simulink model "SHARIEF3IC"  (Simulink 6.6)
settings: Solver=ode45  StartTime=0.0  StopTime=0.01  RelTol=1e-3
libraries: powerlib x10
settings Model: Creator=Y9EE1238  LastModifiedBy=Y9EE1238

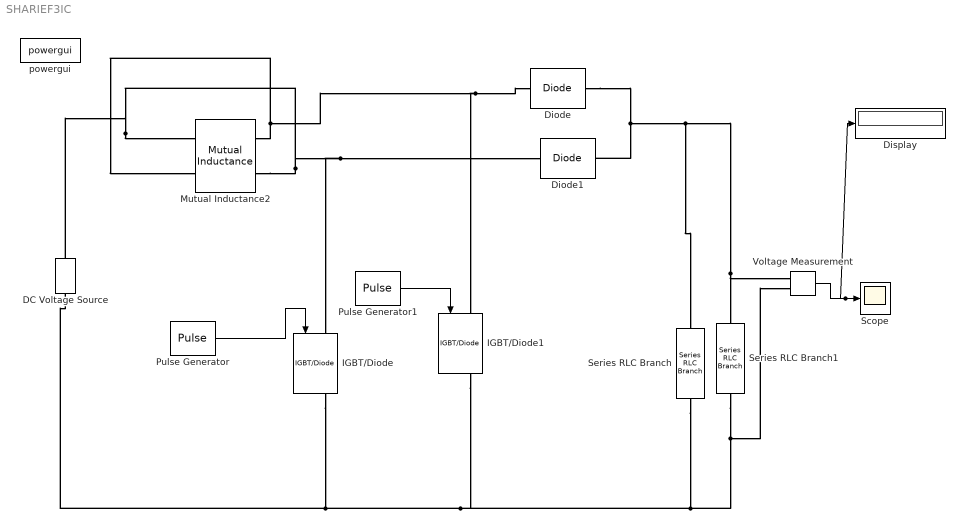
== system SHARIEF3IC ==
  DC Voltage Source : powerlib/Electrical Sources/DC Voltage Source  Orientation=up  DialogController=POWERSYS.PowerSysDialog  SystemSampleTime=-1  Amplitude=20  Measurements=None
  Diode : powerlib/Power Electronics/Diode  DialogController=POWERSYS.PowerSysDialog  SystemSampleTime=-1  Ron=0.001  Lon=0  Vf=0.8  IC=0  Rs=500  Cs=250e-9  Measurements=off
  Diode1 : powerlib/Power Electronics/Diode  DialogController=POWERSYS.PowerSysDialog  SystemSampleTime=-1  Ron=0.001  Lon=0  Vf=0.8  IC=0  Rs=500  Cs=250e-9  Measurements=off
  Display : Display
  IGBT/Diode : powerlib/Power Electronics/IGBT//Diode  Orientation=down  DialogController=POWERSYS.PowerSysDialog  SystemSampleTime=-1  Ron=1e-3  Rs=1e5  Cs=inf  Measurements=on
  IGBT/Diode1 : powerlib/Power Electronics/IGBT//Diode  Orientation=down  DialogController=POWERSYS.PowerSysDialog  SystemSampleTime=-1  Ron=1e-3  Rs=1e5  Cs=inf  Measurements=on
  Mutual Inductance2 : powerlib/Elements/Mutual Inductance  DialogController=POWERSYS.PowerSysDialog  PhysicalDomain=powersysdomain  SubClassName=unknown  LeftPortType=p1  RightPortType=p1  LConnTagsString=a|b  RConnTagsString=A|B  TypeOfMutual=Two or three windings with equal mutual terms  NumberOfWindings=3  SelfImpedance1=[0.0001 6.8e-03]  SelfImpedance2=[0.0001 6.8e-03]  ThreeWindings=off  SelfImpedance3=[ 1.1 1.1e-03]  MutualImpedance=[0.00001 6.3e-03]  InductanceMatrix="[1.0 0.9  0.9 ;  0.9 1.0  0.9;  0.9 0.9 1.0 ] * 1e-3"  ResistanceMatrix="[1.0 0.9  0.9 ;  0.9 1.0  0.9;  0.9 0.9 1.0 ]"  Measurements=None
      settings: AttributesFormatString=\n
  Pulse Generator : DiscretePulseGenerator  PulseType=Time based  Period=0.0005  PulseWidth=50
  Pulse Generator1 : DiscretePulseGenerator  PulseType=Time based  Period=0.0005  PulseWidth=50  PhaseDelay=0.00025
  Scope : Scope
      settings: YMin=0  YMax=45
  Series RLC Branch : powerlib/Elements/Series RLC Branch  Orientation=down  DialogController=POWERSYS.PowerSysDialog  PhysicalDomain=powersysdomain  SubClassName=unknown  LeftPortType=p1  RightPortType=p1  LConnTagsString=__new0  RConnTagsString=__new0  BranchType=C  Resistance=1  Inductance=1e-3  SetiL0=off  InitialCurrent=0  Capacitance=750e-6  Setx0=off  InitialVoltage=0  Measurements=None
  Series RLC Branch1 : powerlib/Elements/Series RLC Branch  Orientation=down  DialogController=POWERSYS.PowerSysDialog  PhysicalDomain=powersysdomain  SubClassName=unknown  LeftPortType=p1  RightPortType=p1  LConnTagsString=__new0  RConnTagsString=__new0  BranchType=R  Resistance=16  Inductance=1e-3  SetiL0=off  InitialCurrent=0  Capacitance=1e-6  Setx0=off  InitialVoltage=0  Measurements=None
  Voltage Measurement : powerlib/Measurements/Voltage Measurement  DialogController=POWERSYS.PowerSysDialog  SystemSampleTime=-1  PhasorSimulation=off  OutputType=Complex  PSBequivalent=0
  powergui : powerlib/powergui  SystemSampleTime=-1  SimulationMode=Discrete  SampleTime=50e-8  echomessages=off  RestoreLinks=warning  x0status=blocks  Frange=[0:2:500]  Ylog=off  Xlog=on  ShowGrid=off  save=off  variable=ZData  ZoomFFT=on  StartTime=0.0  cycles=1  DisplayStyle=1  fundamental=60  FreqAxis=off  MaxFrequency=1000  frequencyindice=0  frequencyindicesteady=1  RmsSteady=1  display=off  Ts=0  frequency=60  methode=off  HookPort=off  Interpol=off
  wires:
  Pulse Generator/1 -> IGBT/Diode/1
  Pulse Generator1/1 -> IGBT/Diode1/1
  Voltage Measurement/1 -> Scope/1, Display/1
  connections:
  Diode/RConn1 -- Diode1/RConn1 -- Series RLC Branch/LConn1 -- Series RLC Branch1/LConn1 -- Voltage Measurement/LConn1
  Series RLC Branch1/RConn1 -- Series RLC Branch/RConn1 -- IGBT/Diode1/RConn1 -- DC Voltage Source/LConn1 -- IGBT/Diode/RConn1 -- Voltage Measurement/LConn2
  Mutual Inductance2/RConn1 -- Mutual Inductance2/LConn2 -- Diode/LConn1 -- IGBT/Diode1/LConn1
  Mutual Inductance2/RConn2 -- Mutual Inductance2/LConn1 -- DC Voltage Source/RConn1 -- Diode1/LConn1 -- IGBT/Diode/LConn1
